simulink model "verify_Battery_EB_mdl"  (R2018b)
settings: Solver=ode45  StartTime=0.0  StopTime=9e5  MaxStep=1  RelTol=1e-3  EnableMultiTasking=on
libraries: carnot x2, simulink x1
settings Model: Creator=drhf  LastModifiedBy=drhf
settings DataIOCC: SaveFormat=Array  SignalLogging=off  DSMLogging=off
settings OptimizationCC: ExpressionDepthLimit=2147483647  LifeSpan=inf
settings DebuggingCC: ArtificialAlgebraicLoopMsg=none  UnderspecifiedInitializationDetection=Classic  MergeDetectMultiDrivingBlocksExec=none  SolverPrmCheckMsg=warning  StateNameClashWarn=warning  SFUnexpectedBacktrackingDiag=warning  SFNoUnconditionalDefaultTransitionDiag=warning  SFExecutionAtInitializationDiag=none
settings HardwareCC: ProdBitPerPointer=32  ProdBitPerSizeT=32  ProdBitPerPtrDiffT=32  ProdLargestAtomicFloat=None  ProdIntDivRoundTo=Undefined  ProdEndianess=Unspecified  ProdWordSize=32  ProdHWDeviceType=32-bit Generic
settings ModelReferenceCC: PropagateSignalLabelsOutOfModel=off
settings SFSimCC: SimUseLocalCustomCode=off
settings RTWCC: RTWUseLocalCustomCode=off
settings CodeAppCC: StateflowObjectComments=on
settings GRTTargetCC: TargetLangStandard=C89/C90 (ANSI)  GeneratePreprocessorConditionals=Disable all  CombineOutputUpdateFcns=off  GRTInterface=on
settings ConfigComp: CovMetricSettings=dw  CovHtmlReporting=on  CovSaveCumulativeToWorkspaceVar=on  CovSaveSingleToWorkspaceVar=on  CovExternalEMLEnable=off

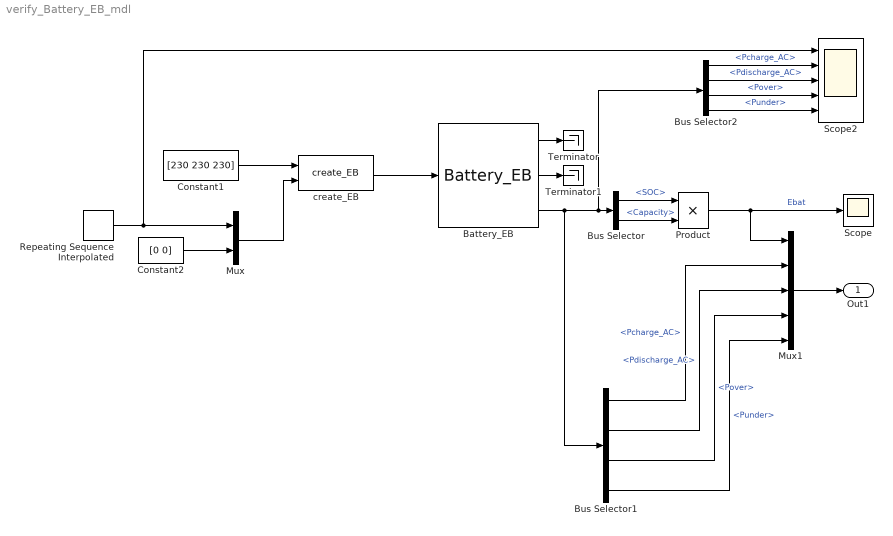
== system verify_Battery_EB_mdl ==
  Battery_EB : carnot/Storage/Electric/Battery_EB  cap_kWh=5e6/3.6e6  eta_ch=0.9  eta_dis=0.9  cap0=1  SOC_max=1  SOC_min=0  Pmax=1000  Pmin=1000  P_standby=10
  Bus Selector : BusSelector  OutputSignals=SOC,Capacity
  Bus Selector1 : BusSelector  OutputSignals=Pcharge_AC,Pdischarge_AC,Pover,Punder
  Bus Selector2 : BusSelector  OutputSignals=Pcharge_AC,Pdischarge_AC,Pover,Punder
  Constant1 : Constant  Value=[230 230 230]
  Constant2 : Constant  Value=[0 0]
  Mux : Mux  Inputs=2
  Mux1 : Mux  Inputs=5
  Product : Product
  Repeating Sequence Interpolated : simulink/Sources/Repeating Sequence Interpolated  OutValues=[0 100 -100 10000 -10000 -10000]  TimeValues=[0 5e5 6e5 7e5 8e5 9e5]  LookUpMeth=Use Input Below  tsamp=1  OutMin=[]  OutMax=[]  OutDataTypeStr=double  OutputDataTypeScalingMode=double  OutDataType=fixdt(0,8)  OutScaling=2^-10
  Scope : Scope
  Scope2 : Scope  NumInputPorts=5
  Terminator : Terminator
  Terminator1 : Terminator
  create_EB : carnot/Source/Simple/create_EB  eID=Power only  f=50  pf1=1  pf2=1  pf3=1
  Out1 : Outport
  wires:
  Constant1/1 -> create_EB/1
  Bus Selector1/3 -> Mux1/4  "<Pover>"
  Bus Selector1/1 -> Mux1/2  "<Pcharge_AC>"
  Product/1 -> Mux1/1, Scope/1  "Ebat"
  Bus Selector1/2 -> Mux1/3  "<Pdischarge_AC>"
  Battery_EB/1 -> Terminator/1
  Bus Selector1/4 -> Mux1/5  "<Punder>"
  create_EB/1 -> Battery_EB/1
  Battery_EB/2 -> Terminator1/1
  Battery_EB/3 -> Bus Selector1/1, Bus Selector2/1, Bus Selector/1
  Bus Selector/1 -> Product/1  "<SOC>"
  Mux/1 -> create_EB/2
  Bus Selector/2 -> Product/2  "<Capacity>"
  Constant2/1 -> Mux/2
  Repeating Sequence Interpolated/1 -> Scope2/1, Mux/1
  Mux1/1 -> Out1/1
  Bus Selector2/1 -> Scope2/2  "<Pcharge_AC>"
  Bus Selector2/2 -> Scope2/3  "<Pdischarge_AC>"
  Bus Selector2/3 -> Scope2/4  "<Pover>"
  Bus Selector2/4 -> Scope2/5  "<Punder>"
